simulink library "StCtrlLibBkRecln"  (R2018b)
settings: Solver=VariableStepAuto  StartTime=0.0  StopTime=10.0  RelTol=1e-3
libraries: simulink x6
settings Model: Creator=sr5w2m  LastModifiedBy=sn55gm

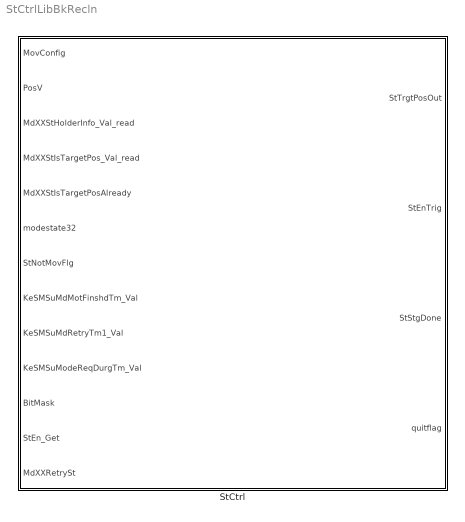
== system StCtrlLibBkRecln ==
  StCtrl : Subsystem

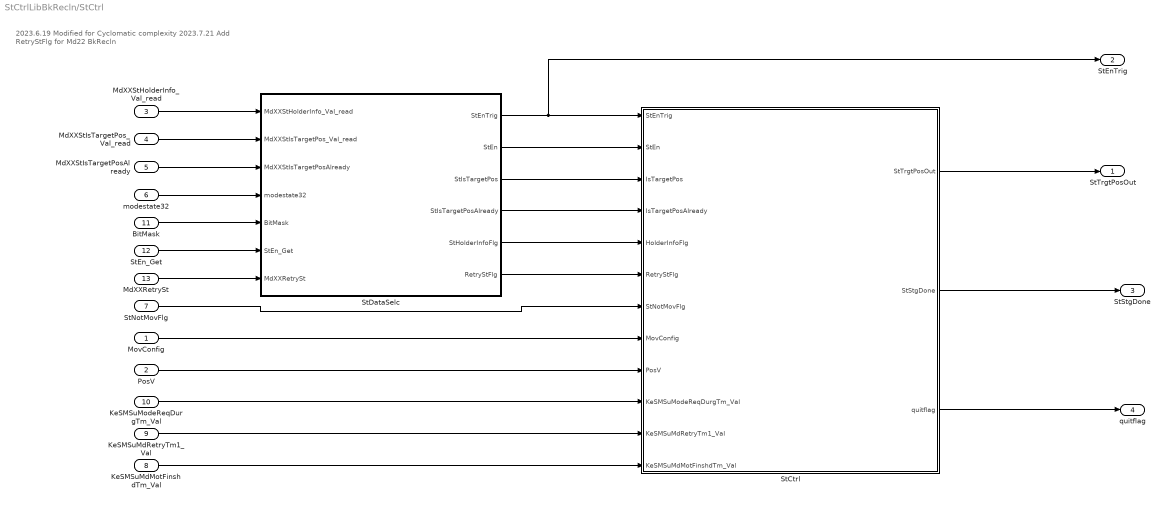
== system StCtrlLibBkRecln/StCtrl ==
  note: 2023.6.19 Modified for Cyclomatic complexity
      | 2023.7.21 Add RetryStFlg for Md22 BkRecln
  MovConfig : Inport
  PosV : Inport  Port=2
  MdXXStHolderInfo_Val_read : Inport  Port=3
  MdXXStIsTargetPos_Val_read : Inport  Port=4
  MdXXStIsTargetPosAlready : Inport  Port=5
  modestate32 : Inport  Port=6
  StNotMovFlg : Inport  Port=7
  KeSMSuMdMotFinshdTm_Val : Inport  Port=8
  KeSMSuMdRetryTm1_Val : Inport  Port=9
  KeSMSuModeReqDurgTm_Val : Inport  Port=10
  BitMask : Inport  Port=11
  StEn_Get : Inport  Port=12
  MdXXRetrySt : Inport  Port=13
  StCtrl : Subsystem
  StDataSelc : Subsystem
  StTrgtPosOut : Outport
  StEnTrig : Outport  Port=2
  StStgDone : Outport  Port=3
  quitflag : Outport  Port=4
  wires:
  StDataSelc/5(StHolderInfoFlg) -> StCtrl/5(HolderInfoFlg)
  MdXXStIsTargetPosAlready/1 -> StDataSelc/3(MdXXStIsTargetPosAlready)
  StDataSelc/1(StEnTrig) -> StEnTrig/1, StCtrl/1(StEnTrig)
  BitMask/1 -> StDataSelc/5(BitMask)
  StDataSelc/2(StEn) -> StCtrl/2(StEn)
  modestate32/1 -> StDataSelc/4(modestate32)
  StDataSelc/3(StIsTargetPos) -> StCtrl/3(IsTargetPos)
  StDataSelc/4(StIsTargetPosAlready) -> StCtrl/4(IsTargetPosAlready)
  MovConfig/1 -> StCtrl/8(MovConfig)
  MdXXStHolderInfo_Val_read/1 -> StDataSelc/1(MdXXStHolderInfo_Val_read)
  MdXXStIsTargetPos_Val_read/1 -> StDataSelc/2(MdXXStIsTargetPos_Val_read)
  KeSMSuModeReqDurgTm_Val/1 -> StCtrl/10(KeSMSuModeReqDurgTm_Val)
  StEn_Get/1 -> StDataSelc/6(StEn_Get)
  StNotMovFlg/1 -> StCtrl/7(StNotMovFlg)
  PosV/1 -> StCtrl/9(PosV)
  StCtrl/2(StStgDone) -> StStgDone/1
  KeSMSuMdRetryTm1_Val/1 -> StCtrl/11(KeSMSuMdRetryTm1_Val)
  KeSMSuMdMotFinshdTm_Val/1 -> StCtrl/12(KeSMSuMdMotFinshdTm_Val)
  StCtrl/1(StTrgtPosOut) -> StTrgtPosOut/1
  StDataSelc/6(RetryStFlg) -> StCtrl/6(RetryStFlg)
  MdXXRetrySt/1 -> StDataSelc/7(MdXXRetrySt)
  StCtrl/3(quitflag) -> quitflag/1

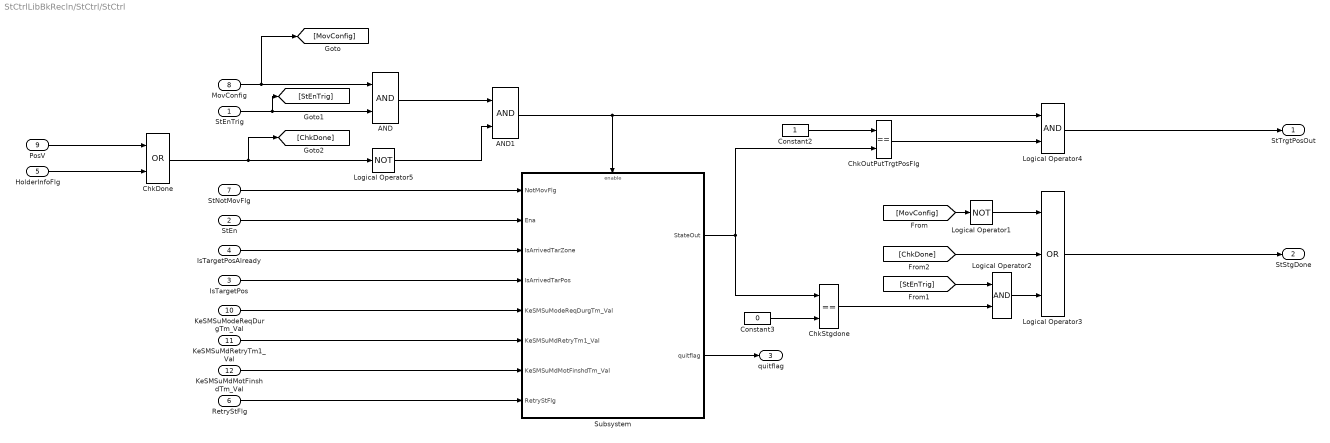
== system StCtrlLibBkRecln/StCtrl/StCtrl ==
  StEnTrig : Inport
  StEn : Inport  Port=2
  IsTargetPos : Inport  Port=3
  IsTargetPosAlready : Inport  Port=4
  HolderInfoFlg : Inport  Port=5
  RetryStFlg : Inport  Port=6
  StNotMovFlg : Inport  Port=7
  MovConfig : Inport  Port=8
  PosV : Inport  Port=9
  KeSMSuModeReqDurgTm_Val : Inport  Port=10
  KeSMSuMdRetryTm1_Val : Inport  Port=11
  KeSMSuMdMotFinshdTm_Val : Inport  Port=12
  AND : Logic  AllPortsSameDT=off  OutDataTypeStr=boolean
  AND1 : Logic  AllPortsSameDT=off  OutDataTypeStr=boolean
  ChkDone : Logic  Operator=OR  AllPortsSameDT=off  OutDataTypeStr=boolean
  ChkOutPutTrgtPosFlg : RelationalOperator  Operator===  OutDataTypeStr=boolean  RndMeth=Simplest
  ChkStgdone : RelationalOperator  Operator===  OutDataTypeStr=boolean  RndMeth=Simplest
  Constant2 : Constant  OutDataTypeStr=uint8
  Constant3 : Constant  Value=0  OutDataTypeStr=uint8
  Logical Operator1 : Logic  Operator=NOT  AllPortsSameDT=off  OutDataTypeStr=boolean
  Logical Operator2 : Logic  AllPortsSameDT=off  OutDataTypeStr=boolean
  Logical Operator3 : Logic  Operator=OR  Inputs=3  AllPortsSameDT=off  OutDataTypeStr=boolean
  Logical Operator4 : Logic  AllPortsSameDT=off  OutDataTypeStr=boolean
  Logical Operator5 : Logic  Operator=NOT  AllPortsSameDT=off  OutDataTypeStr=boolean
  Subsystem : Subsystem
  StTrgtPosOut : Outport
      settings: EnsureOutportIsVirtual=on
  StStgDone : Outport  Port=2
      settings: EnsureOutportIsVirtual=on
  quitflag : Outport  Port=3
  wires:
  StEn/1 -> Subsystem/2(Ena)
  StNotMovFlg/1 -> Subsystem/1(NotMovFlg)
  IsTargetPosAlready/1 -> Subsystem/3(IsArrivedTarZone)
  IsTargetPos/1 -> Subsystem/4(IsArrivedTarPos)
  Logical Operator4/1 -> StTrgtPosOut/1
  Subsystem/1(StateOut) -> ChkStgdone/1, ChkOutPutTrgtPosFlg/2
  StEnTrig/1 -> [StEnTrig], AND/2
  MovConfig/1 -> [MovConfig], AND/1
  Logical Operator3/1 -> StStgDone/1
  [MovConfig] -> Logical Operator1/1
  [StEnTrig] -> Logical Operator2/1
  KeSMSuModeReqDurgTm_Val/1 -> Subsystem/5(KeSMSuModeReqDurgTm_Val)
  KeSMSuMdRetryTm1_Val/1 -> Subsystem/6(KeSMSuMdRetryTm1_Val)
  KeSMSuMdMotFinshdTm_Val/1 -> Subsystem/7(KeSMSuMdMotFinshdTm_Val)
  Constant3/1 -> ChkStgdone/2
  Constant2/1 -> ChkOutPutTrgtPosFlg/1
  ChkStgdone/1 -> Logical Operator2/2
  Logical Operator1/1 -> Logical Operator3/1
  AND1/1 -> Logical Operator4/1, Subsystem/Enable
  ChkOutPutTrgtPosFlg/1 -> Logical Operator4/2
  PosV/1 -> ChkDone/1
  HolderInfoFlg/1 -> ChkDone/2
  ChkDone/1 -> [ChkDone], Logical Operator5/1
  AND/1 -> AND1/1
  Logical Operator5/1 -> AND1/2
  [ChkDone] -> Logical Operator3/2
  Logical Operator2/1 -> Logical Operator3/3
  RetryStFlg/1 -> Subsystem/8(RetryStFlg)
  Subsystem/2(quitflag) -> quitflag/1

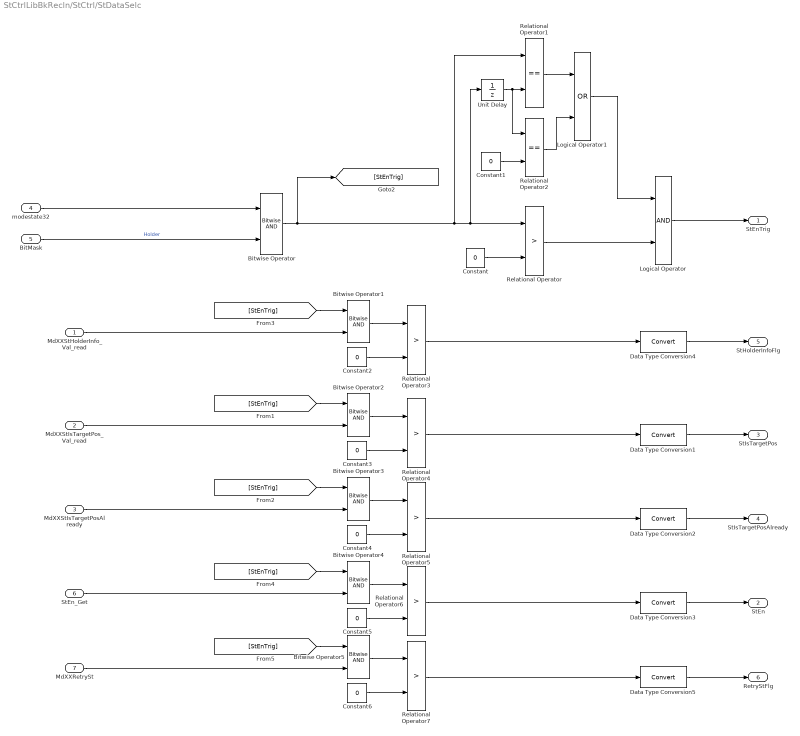
== system StCtrlLibBkRecln/StCtrl/StDataSelc ==
  MdXXStHolderInfo_Val_read : Inport
  MdXXStIsTargetPos_Val_read : Inport  Port=2
  MdXXStIsTargetPosAlready : Inport  Port=3
  modestate32 : Inport  Port=4
  BitMask : Inport  Port=5
  StEn_Get : Inport  Port=6
  MdXXRetrySt : Inport  Port=7
  Bitwise Operator{,1..5} (6 alike) : simulink/Logic and Bit Operations/Bitwise Operator  logicop=AND  UseBitMask=off  NumInputPorts=2  BitMask=bin2dec('11011001')  BitMaskRealWorld=Stored Integer
  Constant{,1..6} (7 alike) : Constant  Value=0  OutDataTypeStr=uint32
  Data Type Conversion{1..5} (5 alike) : DataTypeConversion
  Logical Operator : Logic  AllPortsSameDT=off  OutDataTypeStr=boolean
  Logical Operator1 : Logic  Operator=OR  AllPortsSameDT=off  OutDataTypeStr=boolean
  Relational Operator{,3..7} (6 alike) : RelationalOperator  Operator=>  OutDataTypeStr=boolean  RndMeth=Simplest
  Relational Operator1 : RelationalOperator  Operator===  OutDataTypeStr=boolean  RndMeth=Simplest
  Relational Operator2 : RelationalOperator  Operator===  OutDataTypeStr=boolean  RndMeth=Simplest
  Unit Delay : UnitDelay  SampleTime=-1
  StEnTrig : Outport
      settings: EnsureOutportIsVirtual=on
  StEn : Outport  Port=2
      settings: EnsureOutportIsVirtual=on
  StIsTargetPos : Outport  Port=3
      settings: EnsureOutportIsVirtual=on
  StIsTargetPosAlready : Outport  Port=4
      settings: EnsureOutportIsVirtual=on
  StHolderInfoFlg : Outport  Port=5
      settings: EnsureOutportIsVirtual=on
  RetryStFlg : Outport  Port=6
      settings: EnsureOutportIsVirtual=on
  wires:
  Data Type Conversion4/1 -> StHolderInfoFlg/1
  MdXXStHolderInfo_Val_read/1 -> Bitwise Operator1/2
  Relational Operator2/1 -> Logical Operator1/2
  Relational Operator/1 -> Logical Operator/2
  Constant1/1 -> Relational Operator2/2
  Data Type Conversion2/1 -> StIsTargetPosAlready/1
  Bitwise Operator/1 -> Relational Operator/1, Unit Delay/1, Relational Operator1/1, [StEnTrig]
  Relational Operator3/1 -> Data Type Conversion4/1
  Constant2/1 -> Relational Operator3/2
  [StEnTrig] -> Bitwise Operator1/1
  Data Type Conversion1/1 -> StIsTargetPos/1
  Constant3/1 -> Relational Operator4/2
  Relational Operator4/1 -> Data Type Conversion1/1
  Logical Operator/1 -> StEnTrig/1
  MdXXStIsTargetPosAlready/1 -> Bitwise Operator3/2
  Relational Operator5/1 -> Data Type Conversion2/1
  Bitwise Operator1/1 -> Relational Operator3/1
  [StEnTrig] -> Bitwise Operator3/1
  Unit Delay/1 -> Relational Operator1/2, Relational Operator2/1
  Bitwise Operator3/1 -> Relational Operator5/1
  Bitwise Operator4/1 -> Relational Operator6/1
  [StEnTrig] -> Bitwise Operator4/1
  [StEnTrig] -> Bitwise Operator2/1
  Constant5/1 -> Relational Operator6/2
  MdXXStIsTargetPos_Val_read/1 -> Bitwise Operator2/2
  Logical Operator1/1 -> Logical Operator/1
  Relational Operator6/1 -> Data Type Conversion3/1
  StEn_Get/1 -> Bitwise Operator4/2
  Constant/1 -> Relational Operator/2
  Relational Operator1/1 -> Logical Operator1/1
  Constant4/1 -> Relational Operator5/2
  Bitwise Operator2/1 -> Relational Operator4/1
  Data Type Conversion3/1 -> StEn/1
  modestate32/1 -> Bitwise Operator/1
  BitMask/1 -> Bitwise Operator/2  "Holder"
  MdXXRetrySt/1 -> Bitwise Operator5/2
  Relational Operator7/1 -> Data Type Conversion5/1
  Constant6/1 -> Relational Operator7/2
  Bitwise Operator5/1 -> Relational Operator7/1
  Data Type Conversion5/1 -> RetryStFlg/1
  [StEnTrig] -> Bitwise Operator5/1

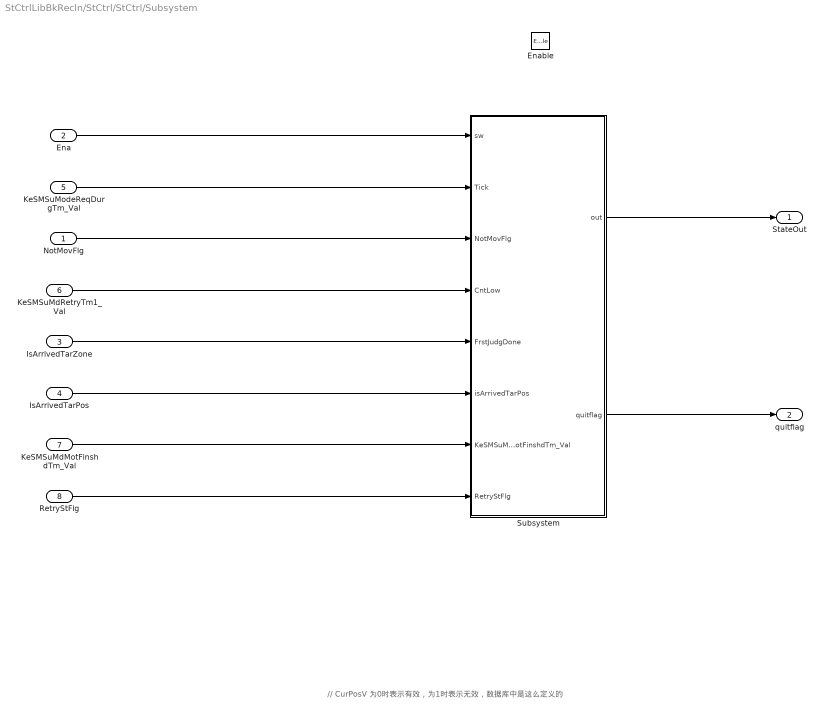
== system StCtrlLibBkRecln/StCtrl/StCtrl/Subsystem ==
  note: // CurPosV 为0时表示有效，为1时表示无效，数据库中是这么定义的
  NotMovFlg : Inport
  Ena : Inport  Port=2
  IsArrivedTarZone : Inport  Port=3
  IsArrivedTarPos : Inport  Port=4
  KeSMSuModeReqDurgTm_Val : Inport  Port=5
  KeSMSuMdRetryTm1_Val : Inport  Port=6
  KeSMSuMdMotFinshdTm_Val : Inport  Port=7
  RetryStFlg : Inport  Port=8
  Enable : EnablePort  StatesWhenEnabling=reset
  Subsystem : Subsystem
  StateOut : Outport
  quitflag : Outport  Port=2
  wires:
  IsArrivedTarPos/1 -> Subsystem/6(isArrivedTarPos)
  IsArrivedTarZone/1 -> Subsystem/5(FrstJudgDone)
  NotMovFlg/1 -> Subsystem/3(NotMovFlg)
  KeSMSuModeReqDurgTm_Val/1 -> Subsystem/2(Tick)
  Ena/1 -> Subsystem/1(sw)
  KeSMSuMdMotFinshdTm_Val/1 -> Subsystem/7(KeSMSuMdMotFinshdTm_Val)
  KeSMSuMdRetryTm1_Val/1 -> Subsystem/4(CntLow)
  Subsystem/1(out) -> StateOut/1
  RetryStFlg/1 -> Subsystem/8(RetryStFlg)
  Subsystem/2(quitflag) -> quitflag/1

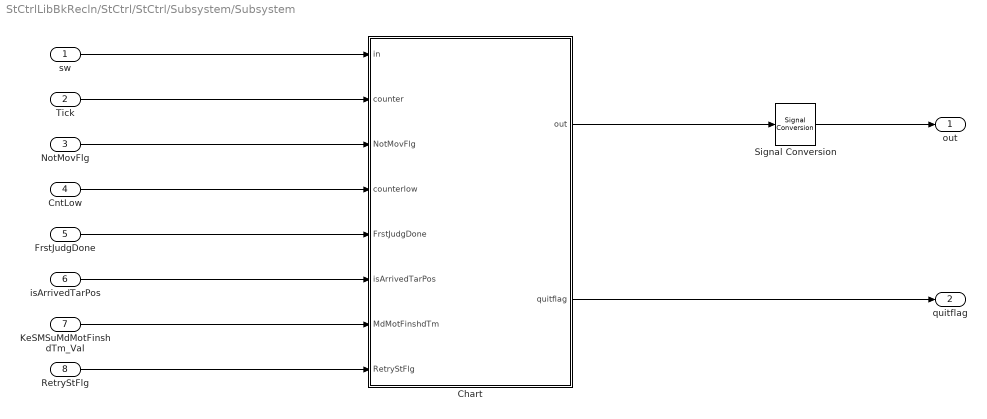
== system StCtrlLibBkRecln/StCtrl/StCtrl/Subsystem/Subsystem ==
  sw : Inport
  Tick : Inport  Port=2
  NotMovFlg : Inport  Port=3
  CntLow : Inport  Port=4
  FrstJudgDone : Inport  Port=5
  isArrivedTarPos : Inport  Port=6
  KeSMSuMdMotFinshdTm_Val : Inport  Port=7
  RetryStFlg : Inport  Port=8
  Chart : Stateflow chart  TreatAsAtomicUnit=on
  Signal Conversion : SignalConversion  OverrideOpt=on
  out : Outport
  quitflag : Outport  Port=2
  wires:
  KeSMSuMdMotFinshdTm_Val/1 -> Chart/7(MdMotFinshdTm)
  Signal Conversion/1 -> out/1
  Tick/1 -> Chart/2(counter)
  FrstJudgDone/1 -> Chart/5(FrstJudgDone)
  isArrivedTarPos/1 -> Chart/6(isArrivedTarPos)
  sw/1 -> Chart/1(in)
  NotMovFlg/1 -> Chart/3(NotMovFlg)
  Chart/1(out) -> Signal Conversion/1
  CntLow/1 -> Chart/4(counterlow)
  RetryStFlg/1 -> Chart/8(RetryStFlg)
  Chart/2(quitflag) -> quitflag/1

== stateflow chart StCtrlLibBkRecln/StCtrl/StCtrl/Subsystem/Subsystem/Chart ==
  state On
    en:TimerOn=0;
    du:TimerOn = TimerOn+1;
    state OutputTargetPos
      en:
      out=1;
      quitflag=0;
      timer=uint16(0);
      du:timer=timer+uint16(1);
      quitflag=0;
    state Reset
      en:
      out=2;
      RetryCnt = RetryCnt+1;
      timer=uint16(1);
      quitflag=1;
      du:
      timer=timer+uint16(1);
      ex:
      quitflag=0;
    OutputTargetPos -> OutputTargetPos [order 1] : [!NotMovFlg]
    (default) -> OutputTargetPos
    OutputTargetPos -> Reset [order 2] : [timer>=counter]
    Reset -> OutputTargetPos : [timer>=counterlow]
  state Done
    en:
    out=0;
    quitflag=0;
  state initial
    en:
    out=2;
    RetryCnt = 0;
    timer=uint16(0);
    quitflag=0;
  (default) -> (junction 48) : {quitflag=0;}
  (junction 48) -> (junction 46) [order 1] : [FrstJudgDone]
  (junction 48) -> initial [order 2]
  (junction 46) -> Done
  initial -> On : [in==true]
  On -> Done [order 2] : [(timer>=MdMotFinshdTm&&isArrivedTarPos)||...
      | TimerOn>=6000||...
      | (timer>=counter&&RetryCnt>=1)]
  On -> initial [order 1] : [in!=true]
  Done -> initial : [RetryStFlg]//2023.7.21 Modefied for Md22 BkRecln
  data: in input; counter input; timer local uint16 size=1; RetryCnt local uint8; out output uint8; NotMovFlg input; counterlow input uint8; FrstJudgDone input boolean; isArrivedTarPos input boolean; MdMotFinshdTm input uint16; TimerOn local uint16 size=1; RetryStFlg input boolean; quitflag output boolean
